simulink library "SimplusGT_2020a"  (R2024b)
settings: Solver=ode45  StartTime=0.0  StopTime=10.0  RelTol=1e-3
undefined symbols (not defined in the file): ang_r, Cf, DiscIntNeverNeededParam, initial, Lc, Lf, m, OtherInputs, P_dc, Sbase, t0, Tm_pu, Ts, V, Vbase, w_droop, w_i, w_pll, w_tau, w_v, Wbase, wc, wfil, x0, Ybase, Zbase
libraries: spsVoltageMeasurementLib x77, spsCurrentMeasurementLib x65, spsControlledCurrentSourceLib x24, spsControlledVoltageSourceLib x19, spsThreePhaseSeriesRLCBranchLib x19, spsSeriesRLCBranchLib x15, spsThreePhaseParallelRLCBranchLib x3, spsThreePhaseBreakerLib x2, $bdroot x1, SimplexPS_2015a x1
(part 5 of 6)

== system SimplusGT_2020a/Grid-Forming Inverter (Simulink Block)/LCL Filter ==
  note: Model for a LCL filter.
      |
      | Author(s): Yitong Li
      |
      | Notes:
      |
      | vi is the converter side voltage, and vg is the grid side voltage.
  Bus Creator : BusCreator  Inputs=5
  "LL -> LN" : Subsystem  AncestorBlock=SimplusGT/LL -> LN
  "LL -> LN1" : Subsystem  AncestorBlock=|
      | SimplusGT/Grid-Forming Inverter
      | (Simulink Block)/LCL Filter/LL -> LN
  Mux{,1..4} (5 alike) : Mux  Inputs=3
  Three-Phase Series RLC Branch : spsThreePhaseSeriesRLCBranchLib/Three-Phase Series RLC Branch  LConnTagsString=A|B|C  RConnTagsString=A|B|C  BranchType=RL  Resistance=Rf  Inductance=Lf  Capacitance=1e-6  Measurements=None
  Three-Phase Series RLC Branch1 : spsThreePhaseSeriesRLCBranchLib/Three-Phase Series RLC Branch  LConnTagsString=A|B|C  RConnTagsString=A|B|C  BranchType=RL  Resistance=Rc  Inductance=Lc  Capacitance=1e-6  Measurements=None
  Three-Phase Series RLC Branch2 : spsThreePhaseSeriesRLCBranchLib/Three-Phase Series RLC Branch  LConnTagsString=A|B|C  RConnTagsString=A|B|C  BranchType=RC  Resistance=Rd  Inductance=Lc  Capacitance=Cf  Measurements=None
  Vab : spsVoltageMeasurementLib/Voltage Measurement  PhasorSimulation=off  OutputType=Complex  PSBequivalent=0
  Vab1 : spsVoltageMeasurementLib/Voltage Measurement  PhasorSimulation=off  OutputType=Complex  PSBequivalent=0
  Vbc : spsVoltageMeasurementLib/Voltage Measurement  PhasorSimulation=off  OutputType=Complex  PSBequivalent=0
  Vbc1 : spsVoltageMeasurementLib/Voltage Measurement  PhasorSimulation=off  OutputType=Complex  PSBequivalent=0
  Vca : spsVoltageMeasurementLib/Voltage Measurement  PhasorSimulation=off  OutputType=Complex  PSBequivalent=0
  Vca1 : spsVoltageMeasurementLib/Voltage Measurement  PhasorSimulation=off  OutputType=Complex  PSBequivalent=0
  iga : spsCurrentMeasurementLib/Current Measurement  PhasorSimulation=off  OutputType=Complex  PSBequivalent=0
  igb : spsCurrentMeasurementLib/Current Measurement  PhasorSimulation=off  OutputType=Complex  PSBequivalent=0
  igc : spsCurrentMeasurementLib/Current Measurement  PhasorSimulation=off  OutputType=Complex  PSBequivalent=0
  ila : spsCurrentMeasurementLib/Current Measurement  PhasorSimulation=off  OutputType=Complex  PSBequivalent=0
  ilb : spsCurrentMeasurementLib/Current Measurement  PhasorSimulation=off  OutputType=Complex  PSBequivalent=0
  ilc : spsCurrentMeasurementLib/Current Measurement  PhasorSimulation=off  OutputType=Complex  PSBequivalent=0
  vca measure : spsVoltageMeasurementLib/Voltage Measurement  PhasorSimulation=off  OutputType=Complex  PSBequivalent=0
  vcb measure : spsVoltageMeasurementLib/Voltage Measurement  PhasorSimulation=off  OutputType=Complex  PSBequivalent=0
  vcc measure : spsVoltageMeasurementLib/Voltage Measurement  PhasorSimulation=off  OutputType=Complex  PSBequivalent=0
  via : PMIOPort  Side=Left
  vib : PMIOPort  Port=2  Side=Left
  vic : PMIOPort  Port=3  Side=Left
  vga : PMIOPort  Port=4  Side=Right
  vgb : PMIOPort  Port=5  Side=Right
  vgc : PMIOPort  Port=6  Side=Right
  N : PMIOPort  Port=7  Side=Left
  m : Outport
  wires:
  [igabc] -> Bus Creator/5  "igabc"
  [ilabc] -> Bus Creator/4  "ilabc"
  [vgabc] -> Bus Creator/3  "vgabc"
  [vcabc] -> Bus Creator/2  "vcabc"
  [viabc] -> Bus Creator/1  "viabc"
  "LL -> LN"/1(Out1) -> [viabc]
  Vab1/1 -> Mux1/1
  Mux1/1 -> "LL -> LN"/1(In1)
  Vca1/1 -> Mux1/3
  Vbc1/1 -> Mux1/2
  Mux3/1 -> [vcabc]
  "LL -> LN1"/1(Out1) -> [vgabc]
  Bus Creator/1 -> m/1
  Mux2/1 -> [ilabc]
  Vbc/1 -> Mux/2
  ilc/1 -> Mux2/3
  Vca/1 -> Mux/3
  iga/1 -> Mux4/1
  igb/1 -> Mux4/2
  vcb measure/1 -> Mux3/2
  vca measure/1 -> Mux3/1
  Mux/1 -> "LL -> LN1"/1(In1)
  Vab/1 -> Mux/1
  vcc measure/1 -> Mux3/3
  igc/1 -> Mux4/3
  ila/1 -> Mux2/1
  ilb/1 -> Mux2/2
  Mux4/1 -> [igabc]
  connections:
  Three-Phase Series RLC Branch/RConn3 -- ilc/LConn1
  Three-Phase Series RLC Branch/RConn2 -- ilb/LConn1
  Three-Phase Series RLC Branch/RConn1 -- ila/LConn1
  Three-Phase Series RLC Branch1/RConn3 -- igc/LConn1
  Three-Phase Series RLC Branch1/RConn1 -- iga/LConn1
  vga/RConn1 -- iga/RConn1 -- Vca/LConn2 -- Vab/LConn1
  Three-Phase Series RLC Branch2/LConn1 -- vca measure/LConn1 -- Three-Phase Series RLC Branch1/LConn1 -- ila/RConn1
  Three-Phase Series RLC Branch2/LConn2 -- vcb measure/LConn1 -- Three-Phase Series RLC Branch1/LConn2 -- ilb/RConn1
  vgb/RConn1 -- igb/RConn1 -- Vab/LConn2 -- Vbc/LConn1
  Three-Phase Series RLC Branch1/RConn2 -- igb/LConn1
  vcc measure/LConn1 -- Three-Phase Series RLC Branch2/LConn3 -- ilc/RConn1 -- Three-Phase Series RLC Branch1/LConn3
  Three-Phase Series RLC Branch/LConn1 -- via/RConn1 -- Vca1/LConn2 -- Vab1/LConn1
  vib/RConn1 -- Vab1/LConn2 -- Vbc1/LConn1 -- Three-Phase Series RLC Branch/LConn2
  Three-Phase Series RLC Branch/LConn3 -- vic/RConn1 -- Vbc1/LConn2 -- Vca1/LConn1
  vgc/RConn1 -- igc/RConn1 -- Vbc/LConn2 -- Vca/LConn1
  vcb measure/LConn2 -- vca measure/LConn2 -- vcc measure/LConn2 -- Three-Phase Series RLC Branch2/RConn3 -- N/RConn1 -- Three-Phase Series RLC Branch2/RConn2 -- Three-Phase Series RLC Branch2/RConn1

== system SimplusGT_2020a/Grid-Forming Inverter (Simulink Block)/P-w droop ==
  note: p-w droop controller
      |
      | Author(s): Yitong Li
      |
      | Notes:
      |
      | The power reference should be in source convention.
  pq : Inport
  Constant : Constant  Value=w0
  Constant2 : Constant  Value=theta0
  Constant4 : Constant  Value=2*pi
  Constant6 : Constant  Value=p0
  Demux : Demux  Outputs=2
  Discrete-Time Integrator : DiscreteIntegrator  SampleTime=Ts  ICPrevOutput=DiscIntNeverNeededParam  ICPrevScaledInput=DiscIntNeverNeededParam
  Filter p : DiscreteTransferFcn  Numerator=w_tau*Ts  Denominator=[1 ((w_tau*Ts)-1)]  SampleTime=Ts
  Gain2 : Gain  Gain=m
  Gain3 : Gain  Gain=Wbase
  Math Function1 : Math  Operator=mod  SignedPower=on
  Sum : Sum
  Sum1 : Sum
  Sum2 : Sum  Inputs=+-
  w : Outport
  theta : Outport  Port=2
  wires:
  Gain3/1 -> Discrete-Time Integrator/1, w/1, [w]
  Sum/1 -> Gain3/1
  Sum2/1 -> Gain2/1
  Constant6/1 -> Sum2/1
  pq/1 -> Demux/1
  Constant4/1 -> Math Function1/2
  Constant/1 -> Sum/2
  Filter p/1 -> Sum2/2
  Discrete-Time Integrator/1 -> Sum1/1
  Gain2/1 -> Sum/1
  Math Function1/1 -> theta/1, [theta]
  Constant2/1 -> [theta0], Sum1/2
  Sum1/1 -> Math Function1/1
  Demux/1 -> Filter p/1  "p"

== system SimplusGT_2020a/Grid-Forming Inverter (Simulink Block)/PQ Calculation (dq-Frame) ==
  note: Power calculation.
      |
      | Author(s): Yitong Li
      |
      | Notes:
      |
      | The calculation is done in dq frame.
  vdq : Inport
  idq : Inport  Port=2
  Mux : Mux  Inputs=2
  Mux1 : Mux  Inputs=2
  P = vd*id+vq*iq : Fcn  Expr=u[1]*u[3]+u[2]*u[4]
  Q = -vd*iq+vq*id : Fcn  Expr=-u[1]*u[4]+u[2]*u[3]
  pq : Outport
  wires:
  Mux/1 -> pq/1
  P = vd*id+vq*iq/1 -> Mux/1
  vdq/1 -> Mux1/1
  idq/1 -> Mux1/2
  Mux1/1 -> P = vd*id+vq*iq/1, Q = -vd*iq+vq*id/1
  Q = -vd*iq+vq*id/1 -> Mux/2

== system SimplusGT_2020a/Grid-Forming Inverter (Simulink Block)/Voltage Controller ==
  vcdq* : Inport
  vcdq : Inport  Port=2
  igdq : Inport  Port=3
  enable : Inport  Port=4
  Constant : Constant  Value=Kcd
  Demux1 : Demux  Outputs=2
  Demux2 : Demux  Outputs=2
  Demux3 : Demux  Outputs=2
  Mux : Mux  Inputs=2
  PI-DT-Estimated d : Subsystem  mask{Kg=Kg, Kp=Kp, Ki=Ki, xmax=xdmax, xmin=-xdmax, Ts=Ts}
      mask prompts: Kg "Estimator Gain"; Kp "Proportional Gain"; Ki "Integral Gain"; xmax "Upper Limit"; xmin "Lower Limit"; Ts "Sampling Time"
  PI-DT-Estimated q : Subsystem  mask{Kg=Kg, Kp=Kp, Ki=Ki, xmax=xqmax, xmin=-xqmax, Ts=Ts}
      mask prompts: Kg "Estimator Gain"; Kp "Proportional Gain"; Ki "Integral Gain"; xmax "Upper Limit"; xmin "Lower Limit"; Ts "Sampling Time"
  Product : Product
  Product1 : Product
  sum_d : Sum  Inputs=+-
  sum_q : Sum
  wCd : Gain  Gain=Wbase*Cf
  wCq : Gain  Gain=Wbase*Cf
  ildq* : Outport
  wires:
  sum_d/1 -> Mux/1
  sum_q/1 -> Mux/2
  vcdq/1 -> Demux1/1
  Demux1/1 -> wCd/1, PI-DT-Estimated d/4(actual)
  Demux1/2 -> PI-DT-Estimated q/1(actual), wCq/1
  Mux/1 -> ildq*/1
  PI-DT-Estimated d/1(Out) -> sum_d/1
  igdq/1 -> Demux3/1
  PI-DT-Estimated q/1(Out) -> sum_q/2
  Demux3/2 -> PI-DT-Estimated q/2(initial)
  Demux3/1 -> PI-DT-Estimated d/3(initial)
  vcdq*/1 -> Demux2/1
  Demux2/1 -> PI-DT-Estimated d/2(reference)
  Demux2/2 -> PI-DT-Estimated q/3(reference)
  enable/1 -> PI-DT-Estimated q/4(enable), PI-DT-Estimated d/1(enable)
  wCd/1 -> Product/1
  Product/1 -> sum_q/1
  wCq/1 -> Product1/2
  Product1/1 -> sum_d/2
  Constant/1 -> Product/2, Product1/1

== system SimplusGT_2020a/Grid-Forming Inverter (Simulink Block)/abc -> dq (Power-Invariant) ==
  note: Frame transformation from abc to dq.
      |
      | Author(s): Yitong Li
      |
      | Notes:
      |
      | The transformation is power-invariant.
      |
      | theta is the angle that d axis leads a axis.
      |
      | q axis leads d axis by 90 degrees.
  abc : Inport
  theta : Inport  Port=2
  ->d : Fcn  Expr=cos(u(4))*u(1) + cos(u(4)-2/3*pi)*u(2) + cos(u(4)-4/3*pi)*u(3)
  ->q : Fcn  Expr=-sin(u(4))*u(1) - sin(u(4)-2/3*pi)*u(2) - sin(u(4)-4/3*pi)*u(3)
  Gain : Gain  Gain=sqrt(2/3)
  Mux5 : Mux  Inputs=2
  Mux6 : Mux  Inputs=2
  dq : Outport
  wires:
  abc/1 -> Gain/1
  ->d/1 -> Mux6/1
  Gain/1 -> Mux5/1
  theta/1 -> Mux5/2
  ->q/1 -> Mux6/2
  Mux6/1 -> dq/1
  Mux5/1 -> ->d/1, ->q/1

== system SimplusGT_2020a/Grid-Forming Inverter (Simulink Block)/abc -> dq (Power-Invariant)1 ==
  note: Frame transformation from abc to dq.
      |
      | Author(s): Yitong Li
      |
      | Notes:
      |
      | The transformation is power-invariant.
      |
      | theta is the angle that d axis leads a axis.
      |
      | q axis leads d axis by 90 degrees.
  abc : Inport
  theta : Inport  Port=2
  ->d : Fcn  Expr=cos(u(4))*u(1) + cos(u(4)-2/3*pi)*u(2) + cos(u(4)-4/3*pi)*u(3)
  ->q : Fcn  Expr=-sin(u(4))*u(1) - sin(u(4)-2/3*pi)*u(2) - sin(u(4)-4/3*pi)*u(3)
  Gain : Gain  Gain=sqrt(2/3)
  Mux5 : Mux  Inputs=2
  Mux6 : Mux  Inputs=2
  dq : Outport
  wires:
  abc/1 -> Gain/1
  ->d/1 -> Mux6/1
  Gain/1 -> Mux5/1
  theta/1 -> Mux5/2
  ->q/1 -> Mux6/2
  Mux6/1 -> dq/1
  Mux5/1 -> ->d/1, ->q/1

== system SimplusGT_2020a/Grid-Forming Inverter (Simulink Block)/abc -> dq (Power-Invariant)2 ==
  note: Frame transformation from abc to dq.
      |
      | Author(s): Yitong Li
      |
      | Notes:
      |
      | The transformation is power-invariant.
      |
      | theta is the angle that d axis leads a axis.
      |
      | q axis leads d axis by 90 degrees.
  abc : Inport
  theta : Inport  Port=2
  ->d : Fcn  Expr=cos(u(4))*u(1) + cos(u(4)-2/3*pi)*u(2) + cos(u(4)-4/3*pi)*u(3)
  ->q : Fcn  Expr=-sin(u(4))*u(1) - sin(u(4)-2/3*pi)*u(2) - sin(u(4)-4/3*pi)*u(3)
  Gain : Gain  Gain=sqrt(2/3)
  Mux5 : Mux  Inputs=2
  Mux6 : Mux  Inputs=2
  dq : Outport
  wires:
  abc/1 -> Gain/1
  ->d/1 -> Mux6/1
  Gain/1 -> Mux5/1
  theta/1 -> Mux5/2
  ->q/1 -> Mux6/2
  Mux6/1 -> dq/1
  Mux5/1 -> ->d/1, ->q/1

== system SimplusGT_2020a/Grid-Forming Inverter (Simulink Block)/dq -> abc (Power-Invariant) ==
  note: Frame transformation from dq to abc.
      |
      | Author(s): Yitong Li
      |
      | Notes:
      |
      | The transformation is power-invariant.
      |
      | theta is the angle that dq axis leads alpha/beta axis, specifically, d axis leads alpha axis.
  dq : Inport
  theta : Inport  Port=2
  ->a : Fcn  Expr=cos(u(3))*u(1) - sin(u(3))*u(2)
  ->b : Fcn  Expr=cos(u(3)-2/3*pi)*u(1) - sin(u(3)-2/3*pi)*u(2)
  ->c : Fcn  Expr=cos(u(3)-4/3*pi)*u(1) - sin(u(3)-4/3*pi)*u(2)
  Gain : Gain  Gain=sqrt(2/3)
  Mux5 : Mux  Inputs=2
  Mux6 : Mux  Inputs=3
  abc : Outport
  wires:
  ->b/1 -> Mux6/2
  ->a/1 -> Mux6/1
  Gain/1 -> Mux5/1
  dq/1 -> Gain/1
  ->c/1 -> Mux6/3
  Mux6/1 -> abc/1
  Mux5/1 -> ->b/1, ->a/1, ->c/1
  theta/1 -> Mux5/2

== system SimplusGT_2020a/Interlink AC-DC (System Object)/PQ Calculation (dq-Frame) ==
  note: Power calculation.
      |
      | Author(s): Yitong Li
      |
      | Notes:
      |
      | The calculation is done in dq frame.
  vdq : Inport
  idq : Inport  Port=2
  Mux : Mux  Inputs=2
  Mux1 : Mux  Inputs=2
  P = vd*id+vq*iq : Fcn  Expr=u[1]*u[3]+u[2]*u[4]
  Q = -vd*iq+vq*id : Fcn  Expr=-u[1]*u[4]+u[2]*u[3]
  pq : Outport
  wires:
  Mux/1 -> pq/1
  P = vd*id+vq*iq/1 -> Mux/1
  vdq/1 -> Mux1/1
  idq/1 -> Mux1/2
  Mux1/1 -> P = vd*id+vq*iq/1, Q = -vd*iq+vq*id/1
  Q = -vd*iq+vq*id/1 -> Mux/2

== system SimplusGT_2020a/Interlink AC-DC (System Object)/abc -> dq (Power-Invariant) ==
  note: Frame transformation from abc to dq.
      |
      | Author(s): Yitong Li
      |
      | Notes:
      |
      | The transformation is power-invariant.
      |
      | theta is the angle that d axis leads a axis.
      |
      | q axis leads d axis by 90 degrees.
  abc : Inport
  theta : Inport  Port=2
  ->d : Fcn  Expr=cos(u(4))*u(1) + cos(u(4)-2/3*pi)*u(2) + cos(u(4)-4/3*pi)*u(3)
  ->q : Fcn  Expr=-sin(u(4))*u(1) - sin(u(4)-2/3*pi)*u(2) - sin(u(4)-4/3*pi)*u(3)
  Gain : Gain  Gain=sqrt(2/3)
  Mux5 : Mux  Inputs=2
  Mux6 : Mux  Inputs=2
  dq : Outport
  wires:
  abc/1 -> Gain/1
  ->d/1 -> Mux6/1
  Gain/1 -> Mux5/1
  theta/1 -> Mux5/2
  ->q/1 -> Mux6/2
  Mux6/1 -> dq/1
  Mux5/1 -> ->d/1, ->q/1

== system SimplusGT_2020a/Interlink AC-DC (System Object)/abc -> dq (Power-Invariant)1 ==
  note: Frame transformation from abc to dq.
      |
      | Author(s): Yitong Li
      |
      | Notes:
      |
      | The transformation is power-invariant.
      |
      | theta is the angle that d axis leads a axis.
      |
      | q axis leads d axis by 90 degrees.
  abc : Inport
  theta : Inport  Port=2
  ->d : Fcn  Expr=cos(u(4))*u(1) + cos(u(4)-2/3*pi)*u(2) + cos(u(4)-4/3*pi)*u(3)
  ->q : Fcn  Expr=-sin(u(4))*u(1) - sin(u(4)-2/3*pi)*u(2) - sin(u(4)-4/3*pi)*u(3)
  Gain : Gain  Gain=sqrt(2/3)
  Mux5 : Mux  Inputs=2
  Mux6 : Mux  Inputs=2
  dq : Outport
  wires:
  abc/1 -> Gain/1
  ->d/1 -> Mux6/1
  Gain/1 -> Mux5/1
  theta/1 -> Mux5/2
  ->q/1 -> Mux6/2
  Mux6/1 -> dq/1
  Mux5/1 -> ->d/1, ->q/1

== system SimplusGT_2020a/Interlink AC-DC (System Object)/dq -> abc (Power-Invariant) ==
  note: Frame transformation from dq to abc.
      |
      | Author(s): Yitong Li
      |
      | Notes:
      |
      | The transformation is power-invariant.
      |
      | theta is the angle that dq axis leads alpha/beta axis, specifically, d axis leads alpha axis.
  dq : Inport
  theta : Inport  Port=2
  ->a : Fcn  Expr=cos(u(3))*u(1) - sin(u(3))*u(2)
  ->b : Fcn  Expr=cos(u(3)-2/3*pi)*u(1) - sin(u(3)-2/3*pi)*u(2)
  ->c : Fcn  Expr=cos(u(3)-4/3*pi)*u(1) - sin(u(3)-4/3*pi)*u(2)
  Gain : Gain  Gain=sqrt(2/3)
  Mux5 : Mux  Inputs=2
  Mux6 : Mux  Inputs=3
  abc : Outport
  wires:
  ->b/1 -> Mux6/2
  ->a/1 -> Mux6/1
  Gain/1 -> Mux5/1
  dq/1 -> Gain/1
  ->c/1 -> Mux6/3
  Mux6/1 -> abc/1
  Mux5/1 -> ->b/1, ->a/1, ->c/1
  theta/1 -> Mux5/2

== system SimplusGT_2020a/L Filter (3ph)/LL -> LN ==
  note: Transformation from line-to-line voltage to line-to-neutral voltage.
      |
      | Author(s): Yitong Li
  In1 : Inport
  Fcn : Fcn  Expr=u[1]-u[3]
  Fcn1 : Fcn  Expr=u[2]-u[1]
  Fcn2 : Fcn  Expr=u[3]-u[2]
  Gain : Gain  Gain=1/3
  Mux9 : Mux  Inputs=3
  Out1 : Outport
  wires:
  In1/1 -> Gain/1
  Gain/1 -> Fcn/1, Fcn1/1, Fcn2/1
  Mux9/1 -> Out1/1
  Fcn2/1 -> Mux9/3
  Fcn1/1 -> Mux9/2
  Fcn/1 -> Mux9/1

== system SimplusGT_2020a/L Filter (3ph)/LL -> LN1 ==
  note: Transformation from line-to-line voltage to line-to-neutral voltage.
      |
      | Author(s): Yitong Li
  In1 : Inport
  Fcn : Fcn  Expr=u[1]-u[3]
  Fcn1 : Fcn  Expr=u[2]-u[1]
  Fcn2 : Fcn  Expr=u[3]-u[2]
  Gain : Gain  Gain=1/3
  Mux9 : Mux  Inputs=3
  Out1 : Outport
  wires:
  In1/1 -> Gain/1
  Gain/1 -> Fcn/1, Fcn1/1, Fcn2/1
  Mux9/1 -> Out1/1
  Fcn2/1 -> Mux9/3
  Fcn1/1 -> Mux9/2
  Fcn/1 -> Mux9/1

== system SimplusGT_2020a/LC Filter (3ph)/LL -> LN ==
  note: Transformation from line-to-line voltage to line-to-neutral voltage.
      |
      | Author(s): Yitong Li
  In1 : Inport
  Fcn : Fcn  Expr=u[1]-u[3]
  Fcn1 : Fcn  Expr=u[2]-u[1]
  Fcn2 : Fcn  Expr=u[3]-u[2]
  Gain : Gain  Gain=1/3
  Mux9 : Mux  Inputs=3
  Out1 : Outport
  wires:
  In1/1 -> Gain/1
  Gain/1 -> Fcn/1, Fcn1/1, Fcn2/1
  Mux9/1 -> Out1/1
  Fcn2/1 -> Mux9/3
  Fcn1/1 -> Mux9/2
  Fcn/1 -> Mux9/1

== system SimplusGT_2020a/LCL Filter (3ph)/LL -> LN ==
  note: Transformation from line-to-line voltage to line-to-neutral voltage.
      |
      | Author(s): Yitong Li
  In1 : Inport
  Fcn : Fcn  Expr=u[1]-u[3]
  Fcn1 : Fcn  Expr=u[2]-u[1]
  Fcn2 : Fcn  Expr=u[3]-u[2]
  Gain : Gain  Gain=1/3
  Mux9 : Mux  Inputs=3
  Out1 : Outport
  wires:
  Fcn/1 -> Mux9/1
  Fcn1/1 -> Mux9/2
  Fcn2/1 -> Mux9/3
  Mux9/1 -> Out1/1
  Gain/1 -> Fcn2/1, Fcn1/1, Fcn/1
  In1/1 -> Gain/1

== system SimplusGT_2020a/LCL Filter (3ph)/LL -> LN1 ==
  note: Transformation from line-to-line voltage to line-to-neutral voltage.
      |
      | Author(s): Yitong Li
  In1 : Inport
  Fcn : Fcn  Expr=u[1]-u[3]
  Fcn1 : Fcn  Expr=u[2]-u[1]
  Fcn2 : Fcn  Expr=u[3]-u[2]
  Gain : Gain  Gain=1/3
  Mux9 : Mux  Inputs=3
  Out1 : Outport
  wires:
  Fcn/1 -> Mux9/1
  Fcn1/1 -> Mux9/2
  Fcn2/1 -> Mux9/3
  Mux9/1 -> Out1/1
  Gain/1 -> Fcn2/1, Fcn1/1, Fcn/1
  In1/1 -> Gain/1

== system SimplusGT_2020a/PLL (vDQ -> vq)/Discrete PI1 ==
  note: Digital PI controller
      |
      | Author(s): Yitong Li
  enable : Inport
  reference : Inport  Port=2
  initial : Inport  Port=3
  actual : Inport  Port=4
  Discrete-Time Integrator : DiscreteIntegrator  gainval=1  ExternalReset=rising  InitialConditionSource=external  InitialCondition=initial  SampleTime=Ts  LimitOutput=on  UpperSaturationLimit=xmax  LowerSaturationLimit=xmin  ICPrevOutput=DiscIntNeverNeededParam  ICPrevScaledInput=DiscIntNeverNeededParam
  Ierror : Sum  Inputs=+-
  Ki : Gain  Gain=Ki  SaturateOnIntegerOverflow=on  OutDataTypeStr=Inherit: Same as input  ParamDataTypeStr=Inherit: Same as input
  Kp : Gain  Gain=Kp  SaturateOnIntegerOverflow=on  OutDataTypeStr=Inherit: Same as input  ParamDataTypeStr=Inherit: Same as input
  Perror : Sum  Inputs=-+
  Product : Product  RndMeth=Zero
  Product1 : Product  RndMeth=Zero
  Saturation : Saturate  UpperLimit=xmax  LowerLimit=xmin
  Sum1 : Sum  SaturateOnIntegerOverflow=on
  Out : Outport
  wires:
  Product1/1 -> Ki/1
  Ierror/1 -> Product1/1
  Product/1 -> Kp/1
  Perror/1 -> Product/1
  actual/1 -> Perror/1, Ierror/2
  reference/1 -> Ierror/1, Perror/2
  initial/1 -> Discrete-Time Integrator/3
  enable/1 -> Product1/2, Product/2, Discrete-Time Integrator/2
  Discrete-Time Integrator/1 -> Sum1/2
  Kp/1 -> Sum1/1
  Ki/1 -> Discrete-Time Integrator/1
  Sum1/1 -> Saturation/1
  Saturation/1 -> Out/1

== system SimplusGT_2020a/PLL (vDQ -> vq)/x1y1 -> x2y2 ==
  note: Frame transformation from x1y1 to x2y2.
      |
      | Author(s): Yitong Li
      |
      | Notes:
      |
      | theta is the phase angle that coordinate 2 (axis) leads coordinate 1 (axis).
  x1y1 : Inport
  theta : Inport  Port=2
  ->x2 : Fcn  Expr=cos(u(3))*u(1) + sin(u(3))*u(2)
  ->y2 : Fcn  Expr=-sin(u(3))*u(1) + cos(u(3))*u(2)
  Mux5 : Mux  Inputs=2
  Mux6 : Mux  Inputs=2
  x2y2 : Outport
  wires:
  ->x2/1 -> Mux6/1
  ->y2/1 -> Mux6/2
  x1y1/1 -> Mux5/1
  theta/1 -> Mux5/2
  Mux5/1 -> ->x2/1, ->y2/1
  Mux6/1 -> x2y2/1

== system SimplusGT_2020a/PLL (vabc -> theta)/Discrete PI ==
  note: Digital PI controller
      |
      | Author(s): Yitong Li
  enable : Inport
  reference : Inport  Port=2
  initial : Inport  Port=3
  actual : Inport  Port=4
  Discrete-Time Integrator : DiscreteIntegrator  gainval=1  ExternalReset=rising  InitialConditionSource=external  InitialCondition=initial  SampleTime=Ts  LimitOutput=on  UpperSaturationLimit=xmax  LowerSaturationLimit=xmin  ICPrevOutput=DiscIntNeverNeededParam  ICPrevScaledInput=DiscIntNeverNeededParam
  Ierror : Sum  Inputs=+-
  Ki : Gain  Gain=Ki  SaturateOnIntegerOverflow=on  OutDataTypeStr=Inherit: Same as input  ParamDataTypeStr=Inherit: Same as input
  Kp : Gain  Gain=Kp  SaturateOnIntegerOverflow=on  OutDataTypeStr=Inherit: Same as input  ParamDataTypeStr=Inherit: Same as input
  Perror : Sum  Inputs=-+
  Product : Product  RndMeth=Zero
  Product1 : Product  RndMeth=Zero
  Saturation : Saturate  UpperLimit=xmax  LowerLimit=xmin
  Sum1 : Sum  SaturateOnIntegerOverflow=on
  Out : Outport
  wires:
  Product1/1 -> Ki/1
  Ierror/1 -> Product1/1
  Product/1 -> Kp/1
  Perror/1 -> Product/1
  actual/1 -> Perror/1, Ierror/2
  reference/1 -> Ierror/1, Perror/2
  initial/1 -> Discrete-Time Integrator/3
  enable/1 -> Product1/2, Product/2, Discrete-Time Integrator/2
  Discrete-Time Integrator/1 -> Sum1/2
  Kp/1 -> Sum1/1
  Ki/1 -> Discrete-Time Integrator/1
  Sum1/1 -> Saturation/1
  Saturation/1 -> Out/1

== system SimplusGT_2020a/PLL (vabc -> theta)/abc -> dq (Power-Invariant) ==
  note: Frame transformation from abc to dq.
      |
      | Author(s): Yitong Li
      |
      | Notes:
      |
      | The transformation is power-invariant.
      |
      | theta is the angle that d axis leads a axis.
      |
      | q axis leads d axis by 90 degrees.
  abc : Inport
  theta : Inport  Port=2
  ->d : Fcn  Expr=cos(u(4))*u(1) + cos(u(4)-2/3*pi)*u(2) + cos(u(4)-4/3*pi)*u(3)
  ->q : Fcn  Expr=-sin(u(4))*u(1) - sin(u(4)-2/3*pi)*u(2) - sin(u(4)-4/3*pi)*u(3)
  Gain : Gain  Gain=sqrt(2/3)
  Mux5 : Mux  Inputs=2
  Mux6 : Mux  Inputs=2
  dq : Outport
  wires:
  abc/1 -> Gain/1
  ->d/1 -> Mux6/1
  Gain/1 -> Mux5/1
  theta/1 -> Mux5/2
  ->q/1 -> Mux6/2
  Mux6/1 -> dq/1
  Mux5/1 -> ->d/1, ->q/1

== system SimplusGT_2020a/PLL (vabc -> vd+jvq)/Discrete PI_d ==
  note: Digital PI controller
      |
      | Author(s): Yitong Li
  enable : Inport
  reference : Inport  Port=2
  initial : Inport  Port=3
  actual : Inport  Port=4
  Discrete-Time Integrator : DiscreteIntegrator  gainval=1  ExternalReset=rising  InitialConditionSource=external  InitialCondition=initial  SampleTime=Ts  LimitOutput=on  UpperSaturationLimit=xmax  LowerSaturationLimit=xmin  ICPrevOutput=DiscIntNeverNeededParam  ICPrevScaledInput=DiscIntNeverNeededParam
  Ierror : Sum  Inputs=+-
  Ki : Gain  Gain=Ki  SaturateOnIntegerOverflow=on  OutDataTypeStr=Inherit: Same as input  ParamDataTypeStr=Inherit: Same as input
  Kp : Gain  Gain=Kp  SaturateOnIntegerOverflow=on  OutDataTypeStr=Inherit: Same as input  ParamDataTypeStr=Inherit: Same as input
  Perror : Sum  Inputs=-+
  Product : Product  RndMeth=Zero
  Product1 : Product  RndMeth=Zero
  Saturation : Saturate  UpperLimit=xmax  LowerLimit=xmin
  Sum1 : Sum  SaturateOnIntegerOverflow=on
  Out : Outport
  wires:
  Product1/1 -> Ki/1
  Ierror/1 -> Product1/1
  Product/1 -> Kp/1
  Perror/1 -> Product/1
  actual/1 -> Perror/1, Ierror/2
  reference/1 -> Ierror/1, Perror/2
  initial/1 -> Discrete-Time Integrator/3
  enable/1 -> Product1/2, Product/2, Discrete-Time Integrator/2
  Discrete-Time Integrator/1 -> Sum1/2
  Kp/1 -> Sum1/1
  Ki/1 -> Discrete-Time Integrator/1
  Sum1/1 -> Saturation/1
  Saturation/1 -> Out/1

== system SimplusGT_2020a/PLL (vabc -> vd+jvq)/Discrete PI_q ==
  note: Digital PI controller
      |
      | Author(s): Yitong Li
  enable : Inport
  reference : Inport  Port=2
  initial : Inport  Port=3
  actual : Inport  Port=4
  Discrete-Time Integrator : DiscreteIntegrator  gainval=1  ExternalReset=rising  InitialConditionSource=external  InitialCondition=initial  SampleTime=Ts  LimitOutput=on  UpperSaturationLimit=xmax  LowerSaturationLimit=xmin  ICPrevOutput=DiscIntNeverNeededParam  ICPrevScaledInput=DiscIntNeverNeededParam
  Ierror : Sum  Inputs=+-
  Ki : Gain  Gain=Ki  SaturateOnIntegerOverflow=on  OutDataTypeStr=Inherit: Same as input  ParamDataTypeStr=Inherit: Same as input
  Kp : Gain  Gain=Kp  SaturateOnIntegerOverflow=on  OutDataTypeStr=Inherit: Same as input  ParamDataTypeStr=Inherit: Same as input
  Perror : Sum  Inputs=-+
  Product : Product  RndMeth=Zero
  Product1 : Product  RndMeth=Zero
  Saturation : Saturate  UpperLimit=xmax  LowerLimit=xmin
  Sum1 : Sum  SaturateOnIntegerOverflow=on
  Out : Outport
  wires:
  Product1/1 -> Ki/1
  Ierror/1 -> Product1/1
  Product/1 -> Kp/1
  Perror/1 -> Product/1
  actual/1 -> Perror/1, Ierror/2
  reference/1 -> Ierror/1, Perror/2
  initial/1 -> Discrete-Time Integrator/3
  enable/1 -> Product1/2, Product/2, Discrete-Time Integrator/2
  Discrete-Time Integrator/1 -> Sum1/2
  Kp/1 -> Sum1/1
  Ki/1 -> Discrete-Time Integrator/1
  Sum1/1 -> Saturation/1
  Saturation/1 -> Out/1

== system SimplusGT_2020a/PLL (vabc -> vd+jvq)/abc -> dq (Power-Invariant) ==
  note: Frame transformation from abc to dq.
      |
      | Author(s): Yitong Li
      |
      | Notes:
      |
      | The transformation is power-invariant.
      |
      | theta is the angle that d axis leads a axis.
      |
      | q axis leads d axis by 90 degrees.
  abc : Inport
  theta : Inport  Port=2
  ->d : Fcn  Expr=cos(u(4))*u(1) + cos(u(4)-2/3*pi)*u(2) + cos(u(4)-4/3*pi)*u(3)
  ->q : Fcn  Expr=-sin(u(4))*u(1) - sin(u(4)-2/3*pi)*u(2) - sin(u(4)-4/3*pi)*u(3)
  Gain : Gain  Gain=sqrt(2/3)
  Mux5 : Mux  Inputs=2
  Mux6 : Mux  Inputs=2
  dq : Outport
  wires:
  abc/1 -> Gain/1
  ->d/1 -> Mux6/1
  Gain/1 -> Mux5/1
  theta/1 -> Mux5/2
  ->q/1 -> Mux6/2
  Mux6/1 -> dq/1
  Mux5/1 -> ->d/1, ->q/1

== system SimplusGT_2020a/PLL (vabc -> vq)/Discrete PI ==
  note: Digital PI controller
      |
      | Author(s): Yitong Li
  enable : Inport
  reference : Inport  Port=2
  initial : Inport  Port=3
  actual : Inport  Port=4
  Discrete-Time Integrator : DiscreteIntegrator  gainval=1  ExternalReset=rising  InitialConditionSource=external  InitialCondition=initial  SampleTime=Ts  LimitOutput=on  UpperSaturationLimit=xmax  LowerSaturationLimit=xmin  ICPrevOutput=DiscIntNeverNeededParam  ICPrevScaledInput=DiscIntNeverNeededParam
  Ierror : Sum  Inputs=+-
  Ki : Gain  Gain=Ki  SaturateOnIntegerOverflow=on  OutDataTypeStr=Inherit: Same as input  ParamDataTypeStr=Inherit: Same as input
  Kp : Gain  Gain=Kp  SaturateOnIntegerOverflow=on  OutDataTypeStr=Inherit: Same as input  ParamDataTypeStr=Inherit: Same as input
  Perror : Sum  Inputs=-+
  Product : Product  RndMeth=Zero
  Product1 : Product  RndMeth=Zero
  Saturation : Saturate  UpperLimit=xmax  LowerLimit=xmin
  Sum1 : Sum  SaturateOnIntegerOverflow=on
  Out : Outport
  wires:
  Product1/1 -> Ki/1
  Ierror/1 -> Product1/1
  Product/1 -> Kp/1
  Perror/1 -> Product/1
  actual/1 -> Perror/1, Ierror/2
  reference/1 -> Ierror/1, Perror/2
  initial/1 -> Discrete-Time Integrator/3
  enable/1 -> Product1/2, Product/2, Discrete-Time Integrator/2
  Discrete-Time Integrator/1 -> Sum1/2
  Kp/1 -> Sum1/1
  Ki/1 -> Discrete-Time Integrator/1
  Sum1/1 -> Saturation/1
  Saturation/1 -> Out/1

== system SimplusGT_2020a/PLL (vabc -> vq)/abc -> dq (Power-Invariant) ==
  note: Frame transformation from abc to dq.
      |
      | Author(s): Yitong Li
      |
      | Notes:
      |
      | The transformation is power-invariant.
      |
      | theta is the angle that d axis leads a axis.
      |
      | q axis leads d axis by 90 degrees.
  abc : Inport
  theta : Inport  Port=2
  ->d : Fcn  Expr=cos(u(4))*u(1) + cos(u(4)-2/3*pi)*u(2) + cos(u(4)-4/3*pi)*u(3)
  ->q : Fcn  Expr=-sin(u(4))*u(1) - sin(u(4)-2/3*pi)*u(2) - sin(u(4)-4/3*pi)*u(3)
  Gain : Gain  Gain=sqrt(2/3)
  Mux5 : Mux  Inputs=2
  Mux6 : Mux  Inputs=2
  dq : Outport
  wires:
  abc/1 -> Gain/1
  ->d/1 -> Mux6/1
  Gain/1 -> Mux5/1
  theta/1 -> Mux5/2
  ->q/1 -> Mux6/2
  Mux6/1 -> dq/1
  Mux5/1 -> ->d/1, ->q/1

== system SimplusGT_2020a/Photovoltaic (dq-Frame System Object)/PQ Calculation (dq-Frame) ==
  note: Power calculation.
      |
      | Author(s): Yitong Li
      |
      | Notes:
      |
      | The calculation is done in dq frame.
  vdq : Inport
  idq : Inport  Port=2
  Mux : Mux  Inputs=2
  Mux1 : Mux  Inputs=2
  P = vd*id+vq*iq : Fcn  Expr=u[1]*u[3]+u[2]*u[4]
  Q = -vd*iq+vq*id : Fcn  Expr=-u[1]*u[4]+u[2]*u[3]
  pq : Outport
  wires:
  Q = -vd*iq+vq*id/1 -> Mux/2
  Mux1/1 -> Q = -vd*iq+vq*id/1, P = vd*id+vq*iq/1
  idq/1 -> Mux1/2
  vdq/1 -> Mux1/1
  P = vd*id+vq*iq/1 -> Mux/1
  Mux/1 -> pq/1

== system SimplusGT_2020a/Photovoltaic (dq-Frame System Object)/abc -> dq (Power-Invariant) ==
  note: Frame transformation from abc to dq.
      |
      | Author(s): Yitong Li
      |
      | Notes:
      |
      | The transformation is power-invariant.
      |
      | theta is the angle that d axis leads a axis.
      |
      | q axis leads d axis by 90 degrees.
  abc : Inport
  theta : Inport  Port=2
  ->d : Fcn  Expr=cos(u(4))*u(1) + cos(u(4)-2/3*pi)*u(2) + cos(u(4)-4/3*pi)*u(3)
  ->q : Fcn  Expr=-sin(u(4))*u(1) - sin(u(4)-2/3*pi)*u(2) - sin(u(4)-4/3*pi)*u(3)
  Gain : Gain  Gain=sqrt(2/3)
  Mux5 : Mux  Inputs=2
  Mux6 : Mux  Inputs=2
  dq : Outport
  wires:
  Mux5/1 -> ->q/1, ->d/1
  Mux6/1 -> dq/1
  ->q/1 -> Mux6/2
  theta/1 -> Mux5/2
  Gain/1 -> Mux5/1
  ->d/1 -> Mux6/1
  abc/1 -> Gain/1

== system SimplusGT_2020a/Photovoltaic (dq-Frame System Object)/abc -> dq (Power-Invariant)1 ==
  note: Frame transformation from abc to dq.
      |
      | Author(s): Yitong Li
      |
      | Notes:
      |
      | The transformation is power-invariant.
      |
      | theta is the angle that d axis leads a axis.
      |
      | q axis leads d axis by 90 degrees.
  abc : Inport
  theta : Inport  Port=2
  ->d : Fcn  Expr=cos(u(4))*u(1) + cos(u(4)-2/3*pi)*u(2) + cos(u(4)-4/3*pi)*u(3)
  ->q : Fcn  Expr=-sin(u(4))*u(1) - sin(u(4)-2/3*pi)*u(2) - sin(u(4)-4/3*pi)*u(3)
  Gain : Gain  Gain=sqrt(2/3)
  Mux5 : Mux  Inputs=2
  Mux6 : Mux  Inputs=2
  dq : Outport
  wires:
  Mux5/1 -> ->q/1, ->d/1
  Mux6/1 -> dq/1
  ->q/1 -> Mux6/2
  theta/1 -> Mux5/2
  Gain/1 -> Mux5/1
  ->d/1 -> Mux6/1
  abc/1 -> Gain/1

== system SimplusGT_2020a/Photovoltaic (dq-Frame System Object)/dq -> abc (Power-Invariant) ==
  note: Frame transformation from dq to abc.
      |
      | Author(s): Yitong Li
      |
      | Notes:
      |
      | The transformation is power-invariant.
      |
      | theta is the angle that dq axis leads alpha/beta axis, specifically, d axis leads alpha axis.
  dq : Inport
  theta : Inport  Port=2
  ->a : Fcn  Expr=cos(u(3))*u(1) - sin(u(3))*u(2)
  ->b : Fcn  Expr=cos(u(3)-2/3*pi)*u(1) - sin(u(3)-2/3*pi)*u(2)
  ->c : Fcn  Expr=cos(u(3)-4/3*pi)*u(1) - sin(u(3)-4/3*pi)*u(2)
  Gain : Gain  Gain=sqrt(2/3)
  Mux5 : Mux  Inputs=2
  Mux6 : Mux  Inputs=3
  abc : Outport
  wires:
  theta/1 -> Mux5/2
  Mux5/1 -> ->c/1, ->a/1, ->b/1
  Mux6/1 -> abc/1
  ->c/1 -> Mux6/3
  dq/1 -> Gain/1
  Gain/1 -> Mux5/1
  ->a/1 -> Mux6/1
  ->b/1 -> Mux6/2

== system SimplusGT_2020a/Synchronous Machine (alpha//beta-Frame) (Simulink Block)/abc -> alpha//beta (Power-Invariant)1 ==
  note: Frame transformation from abc to alpha/beta.
      |
      | Author(s): Yitong Li
      |
      | Notes:
      |
      | The transformation is power-invariant.
  abc : Inport
  ->alpha : Fcn  Expr=u(1) - 1/2*u(2) - 1/2*u(3)
  ->beta : Fcn  Expr=0 + sqrt(3)/2*u(2) - sqrt(3)/2*u(3)
  Gain : Gain  Gain=sqrt(2/3)
  Mux2 : Mux  Inputs=2
  albe : Outport
  wires:
  abc/1 -> Gain/1
  Mux2/1 -> albe/1
  Gain/1 -> ->alpha/1, ->beta/1
  ->alpha/1 -> Mux2/1
  ->beta/1 -> Mux2/2

== system SimplusGT_2020a/Synchronous Machine (alpha//beta-Frame) (Simulink Block)/abc -> alpha//beta (Power-Invariant)2 ==
  note: Frame transformation from abc to alpha/beta.
      |
      | Author(s): Yitong Li
      |
      | Notes:
      |
      | The transformation is power-invariant.
  abc : Inport
  ->alpha : Fcn  Expr=u(1) - 1/2*u(2) - 1/2*u(3)
  ->beta : Fcn  Expr=0 + sqrt(3)/2*u(2) - sqrt(3)/2*u(3)
  Gain : Gain  Gain=sqrt(2/3)
  Mux2 : Mux  Inputs=2
  albe : Outport
  wires:
  abc/1 -> Gain/1
  Mux2/1 -> albe/1
  Gain/1 -> ->alpha/1, ->beta/1
  ->alpha/1 -> Mux2/1
  ->beta/1 -> Mux2/2

== system SimplusGT_2020a/Synchronous Machine (alpha//beta-Frame) (Simulink Block)/alpha//beta -> abc (Power-Invariant)1 ==
  note: Frame transformation from alpha/beta to abc.
      |
      | Author(s): Yitong Li
      |
      | Notes:
      |
      | The transformation is power-invariant.
  albe : Inport
  ->a : Fcn  Expr=u(1) + 0
  ->b : Fcn  Expr=-1/2*u(1) + sqrt(3)/2*u(2)
  ->c : Fcn  Expr=-1/2*u(1) - sqrt(3)/2*u(2)
  Gain : Gain  Gain=sqrt(2/3)
  Mux2 : Mux  Inputs=3
  abc : Outport
  wires:
  Gain/1 -> ->a/1, ->c/1, ->b/1
  Mux2/1 -> abc/1
  ->c/1 -> Mux2/3
  ->b/1 -> Mux2/2
  ->a/1 -> Mux2/1
  albe/1 -> Gain/1

== system SimplusGT_2020a/Synchronous Machine (dq-Frame System Object)/PQ Calculation (dq-Frame) ==
  note: Power calculation.
      |
      | Author(s): Yitong Li
      |
      | Notes:
      |
      | The calculation is done in dq frame.
  vdq : Inport
  idq : Inport  Port=2
  Mux : Mux  Inputs=2
  Mux1 : Mux  Inputs=2
  P = vd*id+vq*iq : Fcn  Expr=u[1]*u[3]+u[2]*u[4]
  Q = -vd*iq+vq*id : Fcn  Expr=-u[1]*u[4]+u[2]*u[3]
  pq : Outport
  wires:
  Q = -vd*iq+vq*id/1 -> Mux/2
  Mux1/1 -> Q = -vd*iq+vq*id/1, P = vd*id+vq*iq/1
  idq/1 -> Mux1/2
  vdq/1 -> Mux1/1
  P = vd*id+vq*iq/1 -> Mux/1
  Mux/1 -> pq/1

== system SimplusGT_2020a/Synchronous Machine (dq-Frame System Object)/abc -> dq (Power-Invariant) ==
  note: Frame transformation from abc to dq.
      |
      | Author(s): Yitong Li
      |
      | Notes:
      |
      | The transformation is power-invariant.
      |
      | theta is the angle that d axis leads a axis.
      |
      | q axis leads d axis by 90 degrees.
  abc : Inport
  theta : Inport  Port=2
  ->d : Fcn  Expr=cos(u(4))*u(1) + cos(u(4)-2/3*pi)*u(2) + cos(u(4)-4/3*pi)*u(3)
  ->q : Fcn  Expr=-sin(u(4))*u(1) - sin(u(4)-2/3*pi)*u(2) - sin(u(4)-4/3*pi)*u(3)
  Gain : Gain  Gain=sqrt(2/3)
  Mux5 : Mux  Inputs=2
  Mux6 : Mux  Inputs=2
  dq : Outport
  wires:
  Mux5/1 -> ->q/1, ->d/1
  Mux6/1 -> dq/1
  ->q/1 -> Mux6/2
  theta/1 -> Mux5/2
  Gain/1 -> Mux5/1
  ->d/1 -> Mux6/1
  abc/1 -> Gain/1

== system SimplusGT_2020a/Synchronous Machine (dq-Frame System Object)/abc -> dq (Power-Invariant)1 ==
  note: Frame transformation from abc to dq.
      |
      | Author(s): Yitong Li
      |
      | Notes:
      |
      | The transformation is power-invariant.
      |
      | theta is the angle that d axis leads a axis.
      |
      | q axis leads d axis by 90 degrees.
  abc : Inport
  theta : Inport  Port=2
  ->d : Fcn  Expr=cos(u(4))*u(1) + cos(u(4)-2/3*pi)*u(2) + cos(u(4)-4/3*pi)*u(3)
  ->q : Fcn  Expr=-sin(u(4))*u(1) - sin(u(4)-2/3*pi)*u(2) - sin(u(4)-4/3*pi)*u(3)
  Gain : Gain  Gain=sqrt(2/3)
  Mux5 : Mux  Inputs=2
  Mux6 : Mux  Inputs=2
  dq : Outport
  wires:
  Mux5/1 -> ->q/1, ->d/1
  Mux6/1 -> dq/1
  ->q/1 -> Mux6/2
  theta/1 -> Mux5/2
  Gain/1 -> Mux5/1
  ->d/1 -> Mux6/1
  abc/1 -> Gain/1

== system SimplusGT_2020a/Synchronous Machine (dq-Frame System Object)/dq -> abc (Power-Invariant) ==
  note: Frame transformation from dq to abc.
      |
      | Author(s): Yitong Li
      |
      | Notes:
      |
      | The transformation is power-invariant.
      |
      | theta is the angle that dq axis leads alpha/beta axis, specifically, d axis leads alpha axis.
  dq : Inport
  theta : Inport  Port=2
  ->a : Fcn  Expr=cos(u(3))*u(1) - sin(u(3))*u(2)
  ->b : Fcn  Expr=cos(u(3)-2/3*pi)*u(1) - sin(u(3)-2/3*pi)*u(2)
  ->c : Fcn  Expr=cos(u(3)-4/3*pi)*u(1) - sin(u(3)-4/3*pi)*u(2)
  Gain : Gain  Gain=sqrt(2/3)
  Mux5 : Mux  Inputs=2
  Mux6 : Mux  Inputs=3
  abc : Outport
  wires:
  theta/1 -> Mux5/2
  Mux5/1 -> ->c/1, ->a/1, ->b/1
  Mux6/1 -> abc/1
  ->c/1 -> Mux6/3
  dq/1 -> Gain/1
  Gain/1 -> Mux5/1
  ->a/1 -> Mux6/1
  ->b/1 -> Mux6/2

== system SimplusGT_2020a/Synchronous Machine (dq-Frame) (Simulink Block)/abc -> dq (Power-Invariant)1 ==
  note: Frame transformation from abc to dq.
      |
      | Author(s): Yitong Li
      |
      | Notes:
      |
      | The transformation is power-invariant.
      |
      | theta is the angle that d axis leads a axis.
      |
      | q axis leads d axis by 90 degrees.
  abc : Inport
  theta : Inport  Port=2
  ->d : Fcn  Expr=cos(u(4))*u(1) + cos(u(4)-2/3*pi)*u(2) + cos(u(4)-4/3*pi)*u(3)
  ->q : Fcn  Expr=-sin(u(4))*u(1) - sin(u(4)-2/3*pi)*u(2) - sin(u(4)-4/3*pi)*u(3)
  Gain : Gain  Gain=sqrt(2/3)
  Mux5 : Mux  Inputs=2
  Mux6 : Mux  Inputs=2
  dq : Outport
  wires:
  Mux5/1 -> ->q/1, ->d/1
  Mux6/1 -> dq/1
  ->q/1 -> Mux6/2
  theta/1 -> Mux5/2
  Gain/1 -> Mux5/1
  ->d/1 -> Mux6/1
  abc/1 -> Gain/1

== system SimplusGT_2020a/Synchronous Machine (dq-Frame) (Simulink Block)/abc -> dq (Power-Invariant)2 ==
  note: Frame transformation from abc to dq.
      |
      | Author(s): Yitong Li
      |
      | Notes:
      |
      | The transformation is power-invariant.
      |
      | theta is the angle that d axis leads a axis.
      |
      | q axis leads d axis by 90 degrees.
  abc : Inport
  theta : Inport  Port=2
  ->d : Fcn  Expr=cos(u(4))*u(1) + cos(u(4)-2/3*pi)*u(2) + cos(u(4)-4/3*pi)*u(3)
  ->q : Fcn  Expr=-sin(u(4))*u(1) - sin(u(4)-2/3*pi)*u(2) - sin(u(4)-4/3*pi)*u(3)
  Gain : Gain  Gain=sqrt(2/3)
  Mux5 : Mux  Inputs=2
  Mux6 : Mux  Inputs=2
  dq : Outport
  wires:
  Mux5/1 -> ->q/1, ->d/1
  Mux6/1 -> dq/1
  ->q/1 -> Mux6/2
  theta/1 -> Mux5/2
  Gain/1 -> Mux5/1
  ->d/1 -> Mux6/1
  abc/1 -> Gain/1

== system SimplusGT_2020a/Synchronous Machine (dq-Frame) (Simulink Block)/dq -> abc (Power-Invariant) ==
  note: Frame transformation from dq to abc.
      |
      | Author(s): Yitong Li
      |
      | Notes:
      |
      | The transformation is power-invariant.
      |
      | theta is the angle that dq axis leads alpha/beta axis, specifically, d axis leads alpha axis.
  dq : Inport
  theta : Inport  Port=2
  ->a : Fcn  Expr=cos(u(3))*u(1) - sin(u(3))*u(2)
  ->b : Fcn  Expr=cos(u(3)-2/3*pi)*u(1) - sin(u(3)-2/3*pi)*u(2)
  ->c : Fcn  Expr=cos(u(3)-4/3*pi)*u(1) - sin(u(3)-4/3*pi)*u(2)
  Gain : Gain  Gain=sqrt(2/3)
  Mux5 : Mux  Inputs=2
  Mux6 : Mux  Inputs=3
  abc : Outport
  wires:
  theta/1 -> Mux5/2
  Mux5/1 -> ->c/1, ->a/1, ->b/1
  Mux6/1 -> abc/1
  ->c/1 -> Mux6/3
  dq/1 -> Gain/1
  Gain/1 -> Mux5/1
  ->a/1 -> Mux6/1
  ->b/1 -> Mux6/2

== system SimplusGT_2020a/Three-Phase Signal/dq -> abc (Power-Invariant) ==
  dq : Inport
  theta : Inport  Port=2
  ->a : Fcn  Expr=cos(u(3))*u(1) - sin(u(3))*u(2)
  ->b : Fcn  Expr=cos(u(3)-2/3*pi)*u(1) - sin(u(3)-2/3*pi)*u(2)
  ->c : Fcn  Expr=cos(u(3)-4/3*pi)*u(1) - sin(u(3)-4/3*pi)*u(2)
  Gain : Gain  Gain=sqrt(2/3)
  Mux5 : Mux  Inputs=2
  Mux6 : Mux  Inputs=3
  abc : Outport
  wires:
  ->b/1 -> Mux6/2
  ->a/1 -> Mux6/1
  Gain/1 -> Mux5/1
  dq/1 -> Gain/1
  ->c/1 -> Mux6/3
  Mux6/1 -> abc/1
  Mux5/1 -> ->b/1, ->a/1, ->c/1
  theta/1 -> Mux5/2

== system SimplusGT_2020a/Grid-Following Inverter (Simulink Block)/Current Controller/PI-DT-Estimated d ==
  enable : Inport
  reference : Inport  Port=2
  initial : Inport  Port=3
  actual : Inport  Port=4
  Discrete-Time Integrator : DiscreteIntegrator  gainval=1  ExternalReset=rising  InitialConditionSource=external  InitialCondition=initial  SampleTime=Ts  LimitOutput=on  UpperSaturationLimit=xmax  LowerSaturationLimit=xmin  ICPrevOutput=DiscIntNeverNeededParam  ICPrevScaledInput=DiscIntNeverNeededParam
  Ierror : Sum  Inputs=+-
  Ki : Gain  Gain=Ki  SaturateOnIntegerOverflow=on  OutDataTypeStr=Inherit: Same as input  ParamDataTypeStr=Inherit: Same as input
  Kp : Gain  Gain=Kp  SaturateOnIntegerOverflow=on  OutDataTypeStr=Inherit: Same as input  ParamDataTypeStr=Inherit: Same as input
  Perror : Sum  Inputs=-+
  Product : Product  RndMeth=Zero
  Product1 : Product  RndMeth=Zero
  Saturation : Saturate  UpperLimit=xmax  LowerLimit=xmin
  Sum1 : Sum  SaturateOnIntegerOverflow=on
  Out : Outport
  wires:
  Saturation/1 -> Out/1
  Sum1/1 -> Saturation/1
  Ki/1 -> Discrete-Time Integrator/1
  Kp/1 -> Sum1/1
  Discrete-Time Integrator/1 -> Sum1/2
  enable/1 -> Discrete-Time Integrator/2, Product/2, Product1/2
  initial/1 -> Discrete-Time Integrator/3
  actual/1 -> Perror/1, Ierror/2
  reference/1 -> Perror/2, Ierror/1
  Perror/1 -> Product/1
  Product/1 -> Kp/1
  Ierror/1 -> Product1/1
  Product1/1 -> Ki/1

== system SimplusGT_2020a/Grid-Following Inverter (Simulink Block)/Current Controller/PI-DT-Estimated q ==
  actual : Inport
  initial : Inport  Port=2
  reference : Inport  Port=3
  enable : Inport  Port=4
  Discrete-Time Integrator : DiscreteIntegrator  gainval=1  ExternalReset=rising  InitialConditionSource=external  InitialCondition=initial  SampleTime=Ts  LimitOutput=on  UpperSaturationLimit=xmax  LowerSaturationLimit=xmin  ICPrevOutput=DiscIntNeverNeededParam  ICPrevScaledInput=DiscIntNeverNeededParam
  Ierror : Sum  Inputs=+-
  Ki : Gain  Gain=Ki  SaturateOnIntegerOverflow=on  OutDataTypeStr=Inherit: Same as input  ParamDataTypeStr=Inherit: Same as input
  Kp : Gain  Gain=Kp  SaturateOnIntegerOverflow=on  OutDataTypeStr=Inherit: Same as input  ParamDataTypeStr=Inherit: Same as input
  Perror : Sum  Inputs=-+
  Product : Product  RndMeth=Zero
  Product1 : Product  RndMeth=Zero
  Saturation : Saturate  UpperLimit=xmax  LowerLimit=xmin
  Sum1 : Sum  SaturateOnIntegerOverflow=on
  Out : Outport
  wires:
  Saturation/1 -> Out/1
  Sum1/1 -> Saturation/1
  Ki/1 -> Discrete-Time Integrator/1
  Kp/1 -> Sum1/1
  Discrete-Time Integrator/1 -> Sum1/2
  enable/1 -> Discrete-Time Integrator/2, Product/2, Product1/2
  initial/1 -> Discrete-Time Integrator/3
  actual/1 -> Ierror/2, Perror/1
  reference/1 -> Perror/2, Ierror/1
  Perror/1 -> Product/1
  Product/1 -> Kp/1
  Ierror/1 -> Product1/1
  Product1/1 -> Ki/1

== system SimplusGT_2020a/Grid-Following Inverter (Simulink Block)/LCL Filter/LL -> LN1 ==
  note: Transformation from line-to-line voltage to line-to-neutral voltage.
      |
      | Author(s): Yitong Li
  In1 : Inport
  Fcn : Fcn  Expr=u[1]-u[3]
  Fcn1 : Fcn  Expr=u[2]-u[1]
  Fcn2 : Fcn  Expr=u[3]-u[2]
  Gain : Gain  Gain=1/3
  Mux9 : Mux  Inputs=3
  Out1 : Outport
  wires:
  Fcn/1 -> Mux9/1
  Fcn1/1 -> Mux9/2
  Fcn2/1 -> Mux9/3
  Mux9/1 -> Out1/1
  Gain/1 -> Fcn2/1, Fcn1/1, Fcn/1
  In1/1 -> Gain/1

== system SimplusGT_2020a/Grid-Following Inverter (Simulink Block)/LCL Filter/LL -> LN2 ==
  note: Transformation from line-to-line voltage to line-to-neutral voltage.
      |
      | Author(s): Yitong Li
  In1 : Inport
  Fcn : Fcn  Expr=u[1]-u[3]
  Fcn1 : Fcn  Expr=u[2]-u[1]
  Fcn2 : Fcn  Expr=u[3]-u[2]
  Gain : Gain  Gain=1/3
  Mux9 : Mux  Inputs=3
  Out1 : Outport
  wires:
  Fcn/1 -> Mux9/1
  Fcn1/1 -> Mux9/2
  Fcn2/1 -> Mux9/3
  Mux9/1 -> Out1/1
  Gain/1 -> Fcn2/1, Fcn1/1, Fcn/1
  In1/1 -> Gain/1

== system SimplusGT_2020a/Grid-Following Inverter (Simulink Block)/PLL (vabc -> vq)/Discrete PI ==
  note: Digital PI controller
      |
      | Author(s): Yitong Li
  enable : Inport
  reference : Inport  Port=2
  initial : Inport  Port=3
  actual : Inport  Port=4
  Discrete-Time Integrator : DiscreteIntegrator  gainval=1  ExternalReset=rising  InitialConditionSource=external  InitialCondition=initial  SampleTime=Ts  LimitOutput=on  UpperSaturationLimit=xmax  LowerSaturationLimit=xmin  ICPrevOutput=DiscIntNeverNeededParam  ICPrevScaledInput=DiscIntNeverNeededParam
  Ierror : Sum  Inputs=+-
  Ki : Gain  Gain=Ki  SaturateOnIntegerOverflow=on  OutDataTypeStr=Inherit: Same as input  ParamDataTypeStr=Inherit: Same as input
  Kp : Gain  Gain=Kp  SaturateOnIntegerOverflow=on  OutDataTypeStr=Inherit: Same as input  ParamDataTypeStr=Inherit: Same as input
  Perror : Sum  Inputs=-+
  Product : Product  RndMeth=Zero
  Product1 : Product  RndMeth=Zero
  Saturation : Saturate  UpperLimit=xmax  LowerLimit=xmin
  Sum1 : Sum  SaturateOnIntegerOverflow=on
  Out : Outport
  wires:
  Saturation/1 -> Out/1
  Sum1/1 -> Saturation/1
  Ki/1 -> Discrete-Time Integrator/1
  Kp/1 -> Sum1/1
  Discrete-Time Integrator/1 -> Sum1/2
  enable/1 -> Discrete-Time Integrator/2, Product/2, Product1/2
  initial/1 -> Discrete-Time Integrator/3
  reference/1 -> Perror/2, Ierror/1
  actual/1 -> Ierror/2, Perror/1
  Perror/1 -> Product/1
  Product/1 -> Kp/1
  Ierror/1 -> Product1/1
  Product1/1 -> Ki/1

== system SimplusGT_2020a/Grid-Following Inverter (Simulink Block)/PLL (vabc -> vq)/abc -> dq (Power-Invariant) ==
  note: Frame transformation from abc to dq.
      |
      | Author(s): Yitong Li
      |
      | Notes:
      |
      | The transformation is power-invariant.
      |
      | theta is the angle that d axis leads a axis.
      |
      | q axis leads d axis by 90 degrees.
  abc : Inport
  theta : Inport  Port=2
  ->d : Fcn  Expr=cos(u(4))*u(1) + cos(u(4)-2/3*pi)*u(2) + cos(u(4)-4/3*pi)*u(3)
  ->q : Fcn  Expr=-sin(u(4))*u(1) - sin(u(4)-2/3*pi)*u(2) - sin(u(4)-4/3*pi)*u(3)
  Gain : Gain  Gain=sqrt(2/3)
  Mux5 : Mux  Inputs=2
  Mux6 : Mux  Inputs=2
  dq : Outport
  wires:
  Mux5/1 -> ->q/1, ->d/1
  Mux6/1 -> dq/1
  ->q/1 -> Mux6/2
  theta/1 -> Mux5/2
  Gain/1 -> Mux5/1
  ->d/1 -> Mux6/1
  abc/1 -> Gain/1

== system SimplusGT_2020a/Grid-Forming Inverter (Simulink Block)/Current Controller/PI-DT-Estimated d ==
  enable : Inport
  reference : Inport  Port=2
  initial : Inport  Port=3
  actual : Inport  Port=4
  Discrete-Time Integrator : DiscreteIntegrator  gainval=1  ExternalReset=rising  InitialConditionSource=external  InitialCondition=initial  SampleTime=Ts  LimitOutput=on  UpperSaturationLimit=xmax  LowerSaturationLimit=xmin  ICPrevOutput=DiscIntNeverNeededParam  ICPrevScaledInput=DiscIntNeverNeededParam
  Ierror : Sum  Inputs=+-
  Ki : Gain  Gain=Ki  SaturateOnIntegerOverflow=on  OutDataTypeStr=Inherit: Same as input  ParamDataTypeStr=Inherit: Same as input
  Kp : Gain  Gain=Kp  SaturateOnIntegerOverflow=on  OutDataTypeStr=Inherit: Same as input  ParamDataTypeStr=Inherit: Same as input
  Perror : Sum  Inputs=-+
  Product : Product  RndMeth=Zero
  Product1 : Product  RndMeth=Zero
  Saturation : Saturate  UpperLimit=xmax  LowerLimit=xmin
  Sum1 : Sum  SaturateOnIntegerOverflow=on
  Out : Outport
  wires:
  Saturation/1 -> Out/1
  Sum1/1 -> Saturation/1
  Ki/1 -> Discrete-Time Integrator/1
  Kp/1 -> Sum1/1
  Discrete-Time Integrator/1 -> Sum1/2
  enable/1 -> Discrete-Time Integrator/2, Product/2, Product1/2
  initial/1 -> Discrete-Time Integrator/3
  actual/1 -> Perror/1, Ierror/2
  reference/1 -> Perror/2, Ierror/1
  Perror/1 -> Product/1
  Product/1 -> Kp/1
  Ierror/1 -> Product1/1
  Product1/1 -> Ki/1

== system SimplusGT_2020a/Grid-Forming Inverter (Simulink Block)/Current Controller/PI-DT-Estimated q ==
  actual : Inport
  initial : Inport  Port=2
  reference : Inport  Port=3
  enable : Inport  Port=4
  Discrete-Time Integrator : DiscreteIntegrator  gainval=1  ExternalReset=rising  InitialConditionSource=external  InitialCondition=initial  SampleTime=Ts  LimitOutput=on  UpperSaturationLimit=xmax  LowerSaturationLimit=xmin  ICPrevOutput=DiscIntNeverNeededParam  ICPrevScaledInput=DiscIntNeverNeededParam
  Ierror : Sum  Inputs=+-
  Ki : Gain  Gain=Ki  SaturateOnIntegerOverflow=on  OutDataTypeStr=Inherit: Same as input  ParamDataTypeStr=Inherit: Same as input
  Kp : Gain  Gain=Kp  SaturateOnIntegerOverflow=on  OutDataTypeStr=Inherit: Same as input  ParamDataTypeStr=Inherit: Same as input
  Perror : Sum  Inputs=-+
  Product : Product  RndMeth=Zero
  Product1 : Product  RndMeth=Zero
  Saturation : Saturate  UpperLimit=xmax  LowerLimit=xmin
  Sum1 : Sum  SaturateOnIntegerOverflow=on
  Out : Outport
  wires:
  Saturation/1 -> Out/1
  Sum1/1 -> Saturation/1
  Ki/1 -> Discrete-Time Integrator/1
  Kp/1 -> Sum1/1
  Discrete-Time Integrator/1 -> Sum1/2
  enable/1 -> Discrete-Time Integrator/2, Product/2, Product1/2
  initial/1 -> Discrete-Time Integrator/3
  actual/1 -> Ierror/2, Perror/1
  reference/1 -> Perror/2, Ierror/1
  Perror/1 -> Product/1
  Product/1 -> Kp/1
  Ierror/1 -> Product1/1
  Product1/1 -> Ki/1

== system SimplusGT_2020a/Grid-Forming Inverter (Simulink Block)/Frequency Droop (iabc -> id)/abc -> dq (Power-Invariant) ==
  note: Frame transformation from abc to dq.
      |
      | Author(s): Yitong Li
      |
      | Notes:
      |
      | The transformation is power-invariant.
      |
      | theta is the angle that d axis leads a axis.
      |
      | q axis leads d axis by 90 degrees.
  abc : Inport
  theta : Inport  Port=2
  ->d : Fcn  Expr=cos(u(4))*u(1) + cos(u(4)-2/3*pi)*u(2) + cos(u(4)-4/3*pi)*u(3)
  ->q : Fcn  Expr=-sin(u(4))*u(1) - sin(u(4)-2/3*pi)*u(2) - sin(u(4)-4/3*pi)*u(3)
  Gain : Gain  Gain=sqrt(2/3)
  Mux5 : Mux  Inputs=2
  Mux6 : Mux  Inputs=2
  dq : Outport
  wires:
  Mux5/1 -> ->q/1, ->d/1
  Mux6/1 -> dq/1
  ->q/1 -> Mux6/2
  theta/1 -> Mux5/2
  Gain/1 -> Mux5/1
  ->d/1 -> Mux6/1
  abc/1 -> Gain/1

== system SimplusGT_2020a/Grid-Forming Inverter (Simulink Block)/LCL Filter/LL -> LN ==
  note: Transformation from line-to-line voltage to line-to-neutral voltage.
      |
      | Author(s): Yitong Li
  In1 : Inport
  Fcn : Fcn  Expr=u[1]-u[3]
  Fcn1 : Fcn  Expr=u[2]-u[1]
  Fcn2 : Fcn  Expr=u[3]-u[2]
  Gain : Gain  Gain=1/3
  Mux9 : Mux  Inputs=3
  Out1 : Outport
  wires:
  Fcn/1 -> Mux9/1
  Fcn1/1 -> Mux9/2
  Fcn2/1 -> Mux9/3
  Mux9/1 -> Out1/1
  Gain/1 -> Fcn2/1, Fcn1/1, Fcn/1
  In1/1 -> Gain/1

== system SimplusGT_2020a/Grid-Forming Inverter (Simulink Block)/LCL Filter/LL -> LN1 ==
  note: Transformation from line-to-line voltage to line-to-neutral voltage.
      |
      | Author(s): Yitong Li
  In1 : Inport
  Fcn : Fcn  Expr=u[1]-u[3]
  Fcn1 : Fcn  Expr=u[2]-u[1]
  Fcn2 : Fcn  Expr=u[3]-u[2]
  Gain : Gain  Gain=1/3
  Mux9 : Mux  Inputs=3
  Out1 : Outport
  wires:
  Fcn/1 -> Mux9/1
  Fcn1/1 -> Mux9/2
  Fcn2/1 -> Mux9/3
  Mux9/1 -> Out1/1
  Gain/1 -> Fcn2/1, Fcn1/1, Fcn/1
  In1/1 -> Gain/1

== system SimplusGT_2020a/Grid-Forming Inverter (Simulink Block)/Voltage Controller/PI-DT-Estimated d ==
  enable : Inport
  reference : Inport  Port=2
  initial : Inport  Port=3
  actual : Inport  Port=4
  Discrete-Time Integrator : DiscreteIntegrator  gainval=1  ExternalReset=rising  InitialConditionSource=external  InitialCondition=initial  SampleTime=Ts  LimitOutput=on  UpperSaturationLimit=xmax  LowerSaturationLimit=xmin  ICPrevOutput=DiscIntNeverNeededParam  ICPrevScaledInput=DiscIntNeverNeededParam
  Ierror : Sum  Inputs=+-
  Ki : Gain  Gain=Ki  SaturateOnIntegerOverflow=on  OutDataTypeStr=Inherit: Same as input  ParamDataTypeStr=Inherit: Same as input
  Kp : Gain  Gain=Kp  SaturateOnIntegerOverflow=on  OutDataTypeStr=Inherit: Same as input  ParamDataTypeStr=Inherit: Same as input
  Perror : Sum  Inputs=-+
  Product : Product  RndMeth=Zero
  Product1 : Product  RndMeth=Zero
  Saturation : Saturate  UpperLimit=xmax  LowerLimit=xmin
  Sum1 : Sum  SaturateOnIntegerOverflow=on
  Out : Outport
  wires:
  Saturation/1 -> Out/1
  Sum1/1 -> Saturation/1
  Ki/1 -> Discrete-Time Integrator/1
  Kp/1 -> Sum1/1
  Discrete-Time Integrator/1 -> Sum1/2
  enable/1 -> Discrete-Time Integrator/2, Product/2, Product1/2
  initial/1 -> Discrete-Time Integrator/3
  actual/1 -> Perror/1, Ierror/2
  reference/1 -> Perror/2, Ierror/1
  Perror/1 -> Product/1
  Product/1 -> Kp/1
  Ierror/1 -> Product1/1
  Product1/1 -> Ki/1
